simulink model "move_to_pose"  (R2020b)
settings: Solver=FixedStepAuto  StartTime=0.0  StopTime=inf  FixedStep=sampleTime  RelTol=1e-3
PreLoadFcn:
  | % Simulation parameters
  | load exampleMap
  | sampleTime = 0.05;
  | 
  | % Robot parameters
  | wheelRadius = 0.05;
  | robotRadius = 0.5;
  | 
  | % Lidar parameters
  | sensorOffset = [0,0];
  | scanAngles = linspace(-pi/2,pi/2,9)';
  | maxRange = 25;
values from neighbouring files (symbols this model uses):
  start = [5,17.5]    [mapgen.m]    (also in path_gen.m = [pose(1) pose(2)])
libraries: mobileRoboticsLib x4, robotalgslib x1, mobileRoboticsTrainingLib x1
settings Model: SimulationMode=accelerator  EnablePacing=on  PacingRate=1000  Creator=scastro  LastModifiedBy=jayas
settings DataIOCC: ReturnWorkspaceOutputs=off
settings DebuggingCC: PregeneratedLibrarySubsystemCodeDiagnostic=none  ArithmeticOperatorsInVariantConditions=warning
settings SFSimCC: SimUseLocalCustomCode=off  CustomCodeUndefinedFunction=UseInterfaceOnly
settings RTWCC: RTWUseLocalCustomCode=off

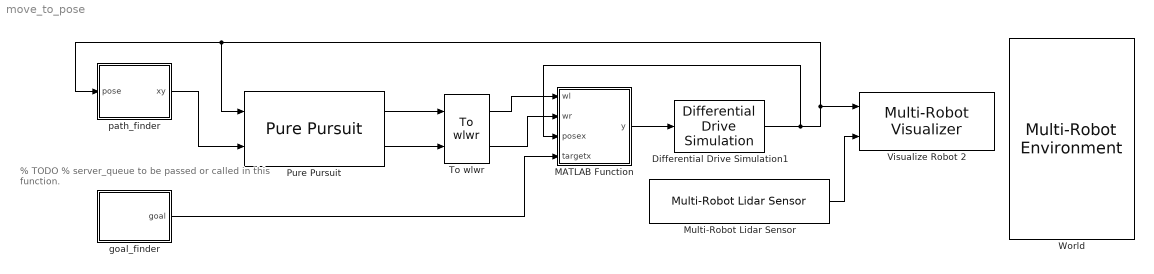
== system move_to_pose ==
  note: % TODO %
      | server_queue to be passed or called in this function.
  Differential Drive Simulation1 : mobileRoboticsLib/Kinematic Models/Differential Drive/Differential Drive Simulation  wheelRadius=wheelRadius  wheelBase=robotRadius  initX=start(1)  initY=start(2)  initAngle=0  Ts=sampleTime
      settings: SourceProductName=Mobile Robotics Simulation Toolbox
  MATLAB Function : MATLAB Function  TreatAsAtomicUnit=on
  Multi-Robot Lidar Sensor : mobileRoboticsLib/Environments/Multi-Robot Lidar Sensor  robotIdx=1  mapName=map  sensorOffset=sensorOffset  scanAngles=scanAngles  maxRange=maxRange
      settings: SourceProductName=Mobile Robotics Simulation Toolbox
  Pure Pursuit : robotalgslib/Pure Pursuit  DesiredLinearVelocity=0.1  MaxAngularVelocity=1  LookaheadDistance=1  TargetDirPort=off  SimulateUsing=Code generation
  To wlwr : mobileRoboticsTrainingLib/To wlwr  axleLength=0.1  wheelR=0.05
  Visualize Robot 2 : mobileRoboticsLib/Environments/Multi-Robot Visualizer  idx=1  radius=robotRadius  robotColor=[1 0 0]  showTraj=off  hasLidar=on  sensorOffset=sensorOffset  scanAngles=scanAngles  maxNumScans=0  hasObjDetector=off  objDetectorOffset=[0,0]  objDetectorAngle=0  objDetectorFOV=pi/2  objDetectorMaxRange=5  hasRobotDetector=off  robotDetectorOffset=sensorOffset  robotDetectorAngle=[pi/2 -pi/2]  robotDetectorFOV=pi  robotDetectorMaxRange=25  robotDetectorNumDetections=0
      link override Goto_ObjDetector: GotoTag=slMultiRobotEnv_ObjDet_2
      link override Goto_RobotDetector: GotoTag=slMultiRobotEnv_RobotDet_2
      settings: SourceProductName=Mobile Robotics Simulation Toolbox
  World : mobileRoboticsLib/Environments/Multi-Robot Environment  numRobots=1  mapName=map  showWaypoints=off  showObjects=off  objectColors=[1 0 0;0 1 0;0 0 1]  objectMarkers='s'  showRobotIds=on  plotSensorLines=on
      settings: SourceProductName=Mobile Robotics Simulation Toolbox
  goal_finder : MATLAB Function  TreatAsAtomicUnit=on
  path_finder : MATLAB Function  TreatAsAtomicUnit=on
  wires:
  Multi-Robot Lidar Sensor/1 -> Visualize Robot 2/2
  Pure Pursuit/2 -> To wlwr/2
  Pure Pursuit/1 -> To wlwr/1
  To wlwr/1 -> MATLAB Function/1(wl)
  To wlwr/2 -> MATLAB Function/2(wr)
  MATLAB Function/1(y) -> Differential Drive Simulation1/1
  Differential Drive Simulation1/1 -> MATLAB Function/3(posex), path_finder/1(pose), Pure Pursuit/1, Visualize Robot 2/1
  goal_finder/1(goal) -> MATLAB Function/4(targetx)
  path_finder/1(xy) -> Pure Pursuit/2

== matlab function move_to_pose/path_finder ==
  data: xy output; pose input
function xy = path_finder(pose)
    xy = path_gen(pose);
end

== matlab function move_to_pose/MATLAB Function ==
  data: wl input; y output; wr input; posex input; targetx input
function y = fcn(wl, wr, posex, targetx)
    if (abs(posex(1) - targetx(1)) < 0.02 && abs(posex(2) - targetx(2)) < 0.02)
        y = [0 0];
    else
        y = [wl, wr];
    end
end

== matlab function move_to_pose/goal_finder ==
  data: goal output
function goal = get_goal()
    server_queue = get_server_queue();
    goal = server_queue.dequeue;
end
